simulink model "modelo_simulacao_Imagens_TCC"  (R2013a)
settings: Solver=ode3  StartTime=0.0  StopTime=1000  FixedStep=0.05  MaxStep=0.1  RelTol=1e-3
undefined symbols (not defined in the file): Dt, Ix, Iy, Iz, Mx, My, Mz, q0, q1, q2, q3, Ref_x, Ref_y, Ref_z, vax, vay, vaz, vnx, vny, vnz, vox, voy, voz, Vsx, Vsy, Vsz, Wx, Wy, Wz, X, Xref, Y, Yref, Z, Zref
libraries: vrlib x4, aerolibutil x3, aerolibtransform2 x2
settings Model: Creator=Daniel  LastModifiedBy=Daniel

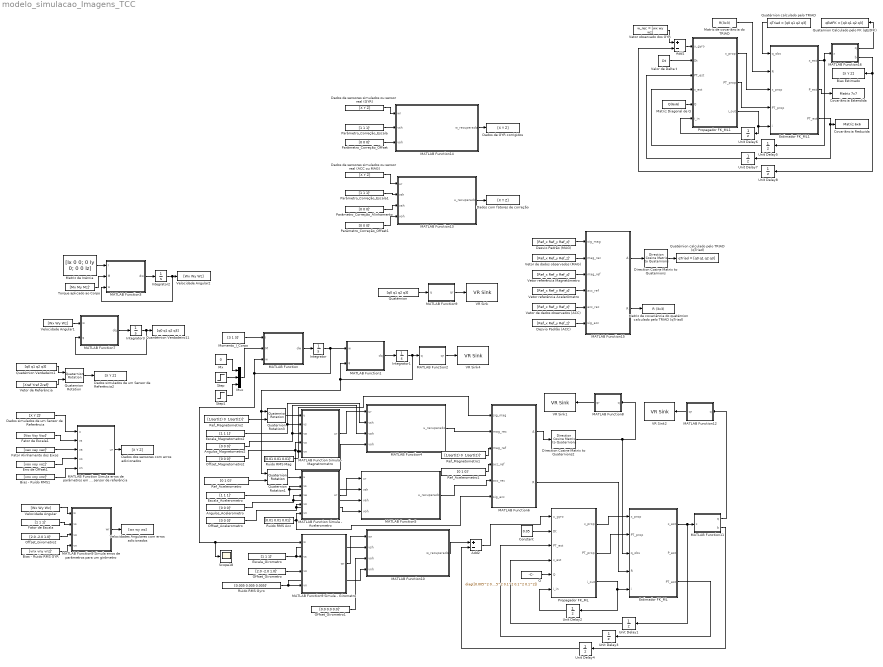
== system modelo_simulacao_Imagens_TCC ==
  Add1 : Sum  Inputs=+-
  Add2 : Sum  Inputs=+-
  Angulos_Acelerometro : Constant  Value=[0 0 0]'
  Angulos_Magnetometro2 : Constant  Value=[0 0 0]'
  Bias - Ruido RMS GYR : Constant  Value=[vnx vny vnz]'
  Bias - Ruído RMS1 : Constant  Value=[vnx vny vnz]'
  Bias Estimado : ToFile  Filename=[X Y Z]  SaveFormat=Timeseries
  Constant : Constant  Value=0.05
  Covariância Estendida : ToFile  Filename=Matriz 7x7  SaveFormat=Timeseries
  Covariância Reduzida : ToFile  Filename=Matriz 6x6  SaveFormat=Timeseries
  Dados com fatores de correção : ToFile  Filename=[X Y Z]  SaveFormat=Timeseries
  Dados de GYR corrigidos : ToFile  Filename=[X Y Z]  SaveFormat=Timeseries
  Dados de sensores simulados ou sensor real (ACC ou MAG) : Constant  Value=[X Y Z]
  Dados de sensores simulados ou sensor real (GYR) : Constant  Value=[X Y Z]
  Dados dos sensores com erros adicionados : ToFile  Filename=[X Y Z]  SaveFormat=Timeseries
  Dados simulados de um Sensor de Referência : Constant  Value=[X Y Z]'
  Dados simulados de um Sensor de Referência2 : ToFile  Filename=[X Y Z]  SaveFormat=Timeseries
  Desvio Padrão (ACC) : Constant  Value=[Ref_x Ref_y Ref_z]'
  Desvio Padrão (MAG) : Constant  Value=[Ref_x Ref_y Ref_z]'
  Direction Cosine Matrix to Quaternions : aerolibtransform2/Direction Cosine Matrix  to Quaternions
  Direction Cosine Matrix to Quaternions2 : aerolibtransform2/Direction Cosine Matrix  to Quaternions
  Erro de Offset1 : Constant  Value=[vox voy voz]'
  Escala_Acelerometro : Constant  Value=[1 1 1]'
  Escala_Girometro : Constant  Value=[1 1 1]'
  Escala_Magnetometro2 : Constant  Value=[1 1 1]'
  Estimador FK_ML : MATLAB Function  TreatAsAtomicUnit=on
  Estimador FK_ML1 : MATLAB Function  TreatAsAtomicUnit=on
  Fator Alinhamento dos Eixos : Constant  Value=[vax vay vaz]'
  Fator de Escala : Constant  Value=[1 1 1]'
  Fator de Escala1 : Constant  Value=[Vsx Vsy Vsz]'
  Integrator : Integrator  InitialCondition=[0 0 0]
  Integrator1 : Integrator  InitialCondition=[1 0 0 0]
  Integrator2 : Integrator  InitialCondition=[0 0 0]
  Integrator3 : Integrator  InitialCondition=[1 0 0 0]
  MATLAB Function : MATLAB Function  TreatAsAtomicUnit=on
  MATLAB Function Simula - Acelerometro : MATLAB Function  TreatAsAtomicUnit=on
  MATLAB Function Simula - Magnetrometro : MATLAB Function  TreatAsAtomicUnit=on
  MATLAB Function Simula erros de parâmetros em um sensor de referência : MATLAB Function  TreatAsAtomicUnit=on
  MATLAB Function1 : MATLAB Function  TreatAsAtomicUnit=on
  MATLAB Function10 : MATLAB Function  TreatAsAtomicUnit=on
  MATLAB Function11 : MATLAB Function  TreatAsAtomicUnit=on
  MATLAB Function12 : MATLAB Function  TreatAsAtomicUnit=on
  MATLAB Function13 : MATLAB Function  TreatAsAtomicUnit=on
  MATLAB Function14 : MATLAB Function  TreatAsAtomicUnit=on
  MATLAB Function15 : MATLAB Function  TreatAsAtomicUnit=on
  MATLAB Function16 : MATLAB Function  TreatAsAtomicUnit=on
  MATLAB Function2 : MATLAB Function  TreatAsAtomicUnit=on
  MATLAB Function3 : MATLAB Function  TreatAsAtomicUnit=on
  MATLAB Function4 : MATLAB Function  TreatAsAtomicUnit=on
  MATLAB Function5 : MATLAB Function  TreatAsAtomicUnit=on
  MATLAB Function6 : MATLAB Function  TreatAsAtomicUnit=on
  MATLAB Function7 : MATLAB Function  TreatAsAtomicUnit=on
  MATLAB Function8 : MATLAB Function  TreatAsAtomicUnit=on
  MATLAB Function9 : MATLAB Function  TreatAsAtomicUnit=on
  MATLAB Function9 Simula - Girometro : MATLAB Function  TreatAsAtomicUnit=on
  MATLAB Function9 Simula erros de parâmetros para um girômetro : MATLAB Function  TreatAsAtomicUnit=on
  Matriz Diagonal de Q : FromFile  FileName=Q(6x6)  SampleTime=0
  Matriz de Inércia : Constant  Value=[Ix 0 0; 0 Iy 0; 0 0 Iz]
  Matriz de covariância do quatérnion calculado pelo TRIAD (qTriad) : ToFile  Filename=R (3x3)  SaveFormat=Timeseries
  Matriz de covariância do TRIAD : FromFile  FileName=R(3x3)  SampleTime=0
  Momento_I_Corpo : Constant  Value=[3 1 3]'
  Mux : Mux  Inputs=3
  Mx : Constant  Value=0
  Offset_Acelerometro : Constant  Value=[0 0 0]'
  Offset_Girometro : Constant  Value=[2.0 -2.0 1.0]'
  Offset_Girometro1 : Constant  Value=[0.0 0.0 0.0]'
  Offset_Girometro2 : Constant  Value=[2.0 -2.0 1.0]'
  Offset_Magnetometro2 : Constant  Value=[0 0 0]'
  Parâmetro_Correção_Alinhamento : Constant  Value=[0 0 0]'
  Parâmetro_Correção_Escala : Constant  Value=[1 1 1]'
  Parâmetro_Correção_Escala1 : Constant  Value=[1 1 1]'
  Parâmetro_Correção_Offset : Constant  Value=[0 0 0]'
  Parâmetro_Correção_Offset1 : Constant  Value=[0 0 0]'
  Propagador FK_ML : MATLAB Function  TreatAsAtomicUnit=on
  Propagador FK_ML1 : MATLAB Function  TreatAsAtomicUnit=on
  Q : Constant  Value=diag([0.005^2 0.005^2 0.005^2 0.1^2 0.1^2 0.1^2])
  Quantérnion Verdadeiro11 : ToFile  Filename=[q0 q1 q2 q3]  SaveFormat=Timeseries
  Quaternion Rotation : aerolibutil/Quaternion Rotation
  Quaternion Rotation1 : aerolibutil/Quaternion Rotation
  Quaternion Rotation3 : aerolibutil/Quaternion Rotation
  Quaternion Calculado pelo FK (qEstFK) : ToFile  Filename=qEstFK = [q0 q1 q2 q3]  SaveFormat=Timeseries
  Quatérnion : Constant  Value=[q0 q1 q2 q3]
  Quatérnion Verdadeiro1 : Constant  Value=[q0 q1 q2 q3]
  Quatérnion calculado pelo TRIAD : FromFile  FileName=qTriad = [q0 q1 q2 q3]  SampleTime=0
  Quatérnion calculado pelo TRIAD (qTriad) : ToFile  Filename=qTriad = [q0 q1 q2 q3]  SaveFormat=Timeseries
  Ref_Acelerometro : Constant  Value=[0 1 0]'
  Ref_Acelerometro1 : Constant  Value=[0 1 0]'
  Ref_Magnetometro1 : Constant  Value="[1/sqrt(2) 0  1/sqrt(2)]'"
  Ref_Magnetometro2 : Constant  Value="[1/sqrt(2) 0  1/sqrt(2)]'"
  Ruido RMS Acc : Constant  Value=[0.01 0.01 0.01]'
  Ruido RMS Gyro : Constant  Value=[0.005 0.005 0.005]'
  Ruido RMS Mag : Constant  Value=[0.01 0.01 0.01]'
  Scope18 : Scope
      settings: YMin=-0.03  YMax=0.12  SaveName=ScopeData18  MaxDataPoints=50000
  Step : Step  Time=.1  Before=5  After=0  SampleTime=0
  Step1 : Step  Time=.1  Before=1  After=0  SampleTime=0
  Torque aplicado ao Corpo : Constant  Value=[Mx My Mz]'
  Unit Delay1 : UnitDelay  InitialCondition=[0 0 0 1 0 0 0]'  SampleTime=-1
  Unit Delay2 : UnitDelay  SampleTime=-1
  Unit Delay3 : UnitDelay  InitialCondition=diag([1 1 1 1 1 1])*1E6  SampleTime=-1
  Unit Delay4 : UnitDelay  InitialCondition=[0 0 0]'  SampleTime=-1
  Unit Delay5 : UnitDelay  InitialCondition=[0 0 0 1 0 0 0]'  SampleTime=-1
  Unit Delay6 : UnitDelay  SampleTime=-1
  Unit Delay7 : UnitDelay  InitialCondition=diag([1 1 1 1 1 1])*1E6  SampleTime=-1
  Unit Delay8 : UnitDelay  InitialCondition=[0 0 0]'  SampleTime=-1
  VR Sink : vrlib/VR Sink  InstantiateOnLoad=on  SampleTime=-1  ViewEnable=on  RemoteChange=off  RemoteView=off  FieldsWritten=H.rotation.4.1.1.double  WorldFileName=C:\Users\Administrator\Desktop\Arquivos WRL\cilindro3.wrl  AutoView=off  VideoDimensions=[]  AllowVariableSize=off
  VR Sink1 : vrlib/VR Sink  InstantiateOnLoad=on  SampleTime=-1  ViewEnable=on  RemoteChange=off  RemoteView=off  FieldsWritten=H.rotation.4.1.1.double  WorldFileName=C:\Users\Administrator\Desktop\Arquivos WRL\cilindro4.wrl  AutoView=off  VideoDimensions=[]  AllowVariableSize=off
  VR Sink2 : vrlib/VR Sink  InstantiateOnLoad=on  SampleTime=-1  ViewEnable=on  RemoteChange=off  RemoteView=off  FieldsWritten=H.rotation.4.1.1.double  WorldFileName=C:\Users\Administrator\Desktop\Arquivos WRL\cilindro5.wrl  AutoView=off  VideoDimensions=[]  AllowVariableSize=off
  VR Sink4 : vrlib/VR Sink  InstantiateOnLoad=on  SampleTime=-1  ViewEnable=on  RemoteChange=off  RemoteView=off  FieldsWritten=H.rotation.4.1.1.double  WorldFileName=C:\Users\Administrator\Desktop\Arquivos WRL\cilindro3.wrl  AutoView=off  VideoDimensions=[]  AllowVariableSize=off
  Valor de Delta t : Constant  Value=Dt
  Velocidade Angular : Constant  Value=[Wx Wy Wz]
  Velocidade Angular1 : Constant  Value=[Wx Wy Wz]
  Velocidade Angular2 : ToFile  Filename=[Wx Wy Wz]  SaveFormat=Timeseries
  Velocidades Angulares com erros adicionados : ToFile  Filename=[wx wy wz]  SaveFormat=Timeseries
  Vetor de Referência : Constant  Value=[Xref Yref Zref]'
  Vetor de dados observados (ACC) : Constant  Value=[Ref_x Ref_y Ref_z]'
  Vetor de dados observados (MAG) : Constant  Value=[Ref_x Ref_y Ref_z]'
  Vetor observado dos GYR : FromFile  FileName=w_rec = [wx wy wz]  SampleTime=0
  Vetor referência Acelerômetro : Constant  Value=[Ref_x Ref_y Ref_z]'
  Vetor referência Magnetômetro : Constant  Value=[Ref_x Ref_y Ref_z]'
  wires:
  Momento_I_Corpo/1 -> MATLAB Function/1(I)
  Mux/1 -> MATLAB Function/2(M)
  Mx/1 -> Mux/1
  Step/1 -> Mux/2
  Step1/1 -> Mux/3
  MATLAB Function/1(dw) -> Integrator/1
  Integrator/1 -> MATLAB Function1/1(w), MATLAB Function/3(w), Scope18/1, MATLAB Function9 Simula - Girometro/1(w)
  MATLAB Function1/1(dq) -> Integrator1/1
  MATLAB Function2/1(qr) -> VR Sink4/1
  Quaternion Rotation3/1 -> MATLAB Function Simula - Magnetrometro/1(u)
  Quaternion Rotation1/1 -> MATLAB Function Simula - Acelerometro/1(u)
  Ref_Magnetometro2/1 -> Quaternion Rotation3/2
  Ref_Acelerometro/1 -> Quaternion Rotation1/2
  Ruido RMS Mag/1 -> MATLAB Function6/1(sig_mag), MATLAB Function Simula - Magnetrometro/5(vn)
  Ruido RMS Acc/1 -> MATLAB Function Simula - Acelerometro/5(vn), MATLAB Function6/6(sig_acc)
  Offset_Magnetometro2/1 -> MATLAB Function Simula - Magnetrometro/4(vo), MATLAB Function4/4(voh)
  Escala_Acelerometro/1 -> MATLAB Function Simula - Acelerometro/2(vs), MATLAB Function5/2(vsh)
  Angulos_Acelerometro/1 -> MATLAB Function Simula - Acelerometro/3(va), MATLAB Function5/3(vah)
  Offset_Acelerometro/1 -> MATLAB Function Simula - Acelerometro/4(vo), MATLAB Function5/4(voh)
  MATLAB Function Simula - Magnetrometro/1(ur) -> MATLAB Function4/1(ur)
  MATLAB Function Simula - Acelerometro/1(ur) -> MATLAB Function5/1(ur)
  Escala_Magnetometro2/1 -> MATLAB Function Simula - Magnetrometro/2(vs), MATLAB Function4/2(vsh)
  Angulos_Magnetometro2/1 -> MATLAB Function Simula - Magnetrometro/3(va), MATLAB Function4/3(vah)
  MATLAB Function5/1(u_recuperado) -> MATLAB Function6/5(acc_rec)
  MATLAB Function4/1(u_recuperado) -> MATLAB Function6/2(mag_rec)
  Ref_Magnetometro1/1 -> MATLAB Function6/3(mag_ref)
  Ref_Acelerometro1/1 -> MATLAB Function6/4(acc_ref)
  MATLAB Function6/1(A) -> Direction Cosine Matrix to Quaternions2/1
  MATLAB Function8/1(qr) -> VR Sink1/1
  MATLAB Function9 Simula - Girometro/1(wr) -> MATLAB Function10/1(wr)
  Escala_Girometro/1 -> MATLAB Function10/2(vsh), MATLAB Function9 Simula - Girometro/2(vs)
  Offset_Girometro/1 -> MATLAB Function9 Simula - Girometro/3(vo)
  Ruido RMS Gyro/1 -> MATLAB Function10/4(vnh), MATLAB Function9 Simula - Girometro/4(vn)
  Offset_Girometro1/1 -> MATLAB Function10/3(voh)
  Propagador FK_ML/1(x_prop) -> Estimador FK_ML/1(x_prop)
  Propagador FK_ML/3(i_out) -> Unit Delay2/1, Estimador FK_ML/5(i)
  Unit Delay2/1 -> Propagador FK_ML/6(i_in)
  Q/1 -> Propagador FK_ML/5(Q)
  Constant/1 -> Propagador FK_ML/2(Dt)
  MATLAB Function10/1(w_recuperado) -> Add2/1
  MATLAB Function6/2(R) -> Estimador FK_ML/4(R)
  Estimador FK_ML/3(PT_est) -> Unit Delay3/1
  Unit Delay1/1 -> Propagador FK_ML/4(x_est)
  Unit Delay3/1 -> Propagador FK_ML/3(PT_est)
  Propagador FK_ML/2(PT_prop) -> Estimador FK_ML/2(PT_prop)
  Direction Cosine Matrix to Quaternions2/1 -> MATLAB Function8/1(q), Estimador FK_ML/3(q_obs)
  Integrator1/1 -> Quaternion Rotation3/1, Quaternion Rotation1/1, MATLAB Function1/2(q), MATLAB Function2/1(q)
  Estimador FK_ML/1(x_est) -> Unit Delay1/1, MATLAB Function11/1(x)
  Add2/1 -> Propagador FK_ML/1(u_gyro)
  MATLAB Function11/2(b) -> Unit Delay4/1
  Unit Delay4/1 -> Add2/2
  MATLAB Function12/1(qr) -> VR Sink2/1
  MATLAB Function11/1(q) -> MATLAB Function12/1(q)
  MATLAB Function3/1(dw) -> Integrator2/1
  Integrator2/1 -> Velocidade Angular2/1, MATLAB Function3/3(w)
  Matriz de Inércia/1 -> MATLAB Function3/1(I)
  Torque aplicado ao Corpo/1 -> MATLAB Function3/2(M)
  MATLAB Function7/1(dq) -> Integrator3/1
  Integrator3/1 -> Quantérnion Verdadeiro11/1, MATLAB Function7/2(q)
  Velocidade Angular1/1 -> MATLAB Function7/1(w)
  Vetor de Referência/1 -> Quaternion Rotation/2
  Quatérnion Verdadeiro1/1 -> Quaternion Rotation/1
  Quaternion Rotation/1 -> Dados simulados de um Sensor de Referência2/1
  Fator de Escala1/1 -> MATLAB Function Simula erros de parâmetros em um sensor de referência/2(vs)
  Fator Alinhamento dos Eixos/1 -> MATLAB Function Simula erros de parâmetros em um sensor de referência/3(va)
  Erro de Offset1/1 -> MATLAB Function Simula erros de parâmetros em um sensor de referência/4(vo)
  Bias - Ruído RMS1/1 -> MATLAB Function Simula erros de parâmetros em um sensor de referência/5(vn)
  Dados simulados de um Sensor de Referência/1 -> MATLAB Function Simula erros de parâmetros em um sensor de referência/1(u)
  MATLAB Function Simula erros de parâmetros em um sensor de referência/1(ur) -> Dados dos sensores com erros adicionados/1
  Bias - Ruido RMS GYR/1 -> MATLAB Function9 Simula erros de parâmetros para um girômetro/4(vn)
  Fator de Escala/1 -> MATLAB Function9 Simula erros de parâmetros para um girômetro/2(vs)
  Offset_Girometro2/1 -> MATLAB Function9 Simula erros de parâmetros para um girômetro/3(vo)
  MATLAB Function9 Simula erros de parâmetros para um girômetro/1(wr) -> Velocidades Angulares com erros adicionados/1
  Velocidade Angular/1 -> MATLAB Function9 Simula erros de parâmetros para um girômetro/1(w)
  MATLAB Function9/1(qr) -> VR Sink/1
  Quatérnion/1 -> MATLAB Function9/1(q)
  Parâmetro_Correção_Escala1/1 -> MATLAB Function13/2(vsh)
  Parâmetro_Correção_Alinhamento/1 -> MATLAB Function13/3(vah)
  Parâmetro_Correção_Offset1/1 -> MATLAB Function13/4(voh)
  Dados de sensores simulados ou sensor real (ACC ou MAG)/1 -> MATLAB Function13/1(ur)
  MATLAB Function13/1(u_recuperado) -> Dados com fatores de correção/1
  MATLAB Function14/1(w_recuperado) -> Dados de GYR corrigidos/1
  Parâmetro_Correção_Offset/1 -> MATLAB Function14/3(voh)
  Parâmetro_Correção_Escala/1 -> MATLAB Function14/2(vsh)
  Dados de sensores simulados ou sensor real (GYR)/1 -> MATLAB Function14/1(wr)
  MATLAB Function15/1(A) -> Direction Cosine Matrix to Quaternions/1
  Vetor referência Acelerômetro/1 -> MATLAB Function15/4(acc_ref)
  Vetor referência Magnetômetro/1 -> MATLAB Function15/3(mag_ref)
  Vetor de dados observados (ACC)/1 -> MATLAB Function15/5(acc_rec)
  Desvio Padrão (ACC)/1 -> MATLAB Function15/6(sig_acc)
  Desvio Padrão (MAG)/1 -> MATLAB Function15/1(sig_mag)
  Vetor de dados observados (MAG)/1 -> MATLAB Function15/2(mag_rec)
  Direction Cosine Matrix to Quaternions/1 -> Quatérnion calculado pelo TRIAD (qTriad)/1
  MATLAB Function15/2(R) -> Matriz de covariância do quatérnion calculado pelo TRIAD (qTriad)/1
  Propagador FK_ML1/1(x_prop) -> Estimador FK_ML1/3(x_prop)
  Propagador FK_ML1/3(i_out) -> Unit Delay6/1, Estimador FK_ML1/5(i)
  Unit Delay6/1 -> Propagador FK_ML1/6(i_in)
  Valor de Delta t/1 -> Propagador FK_ML1/2(Dt)
  Estimador FK_ML1/3(PT_est) -> Covariância Reduzida/1, Unit Delay7/1
  Unit Delay5/1 -> Propagador FK_ML1/4(x_est)
  Unit Delay7/1 -> Propagador FK_ML1/3(PT_est)
  Propagador FK_ML1/2(PT_prop) -> Estimador FK_ML1/4(PT_prop)
  Estimador FK_ML1/1(x_est) -> MATLAB Function16/1(x), Unit Delay5/1
  Add1/1 -> Propagador FK_ML1/1(u_gyro)
  MATLAB Function16/2(b) -> Bias Estimado/1, Unit Delay8/1
  Unit Delay8/1 -> Add1/2
  MATLAB Function16/1(q) -> Quaternion Calculado pelo FK (qEstFK)/1
  Estimador FK_ML1/2(P_est) -> Covariância Estendida/1
  Matriz Diagonal de Q/1 -> Propagador FK_ML1/5(Q)
  Matriz de covariância do TRIAD/1 -> Estimador FK_ML1/2(R)
  Quatérnion calculado pelo TRIAD/1 -> Estimador FK_ML1/1(q_obs)
  Vetor observado dos GYR/1 -> Add1/1

== matlab function modelo_simulacao_Imagens_TCC/MATLAB Function1 ==
  data: w input; dq output; q input
function dq = cinematica(w,q)
%#eml
wx = w(1);
wy = w(2);
wz = w(3);

q = q/norm(q);

qteta = q(1);
qx = q(2);
qy = q(3);
qz = q(4);

W = [0 -wx -wy -wz; wx 0 wz -wy; wy -wz 0 wx; wz wy -wx 0];
%W=[0 wz -wy wx; -wz 0 wx wy; wy -wx 0 wz; -wx -wy -wz 0];
dq=0.5*W*[qteta qx qy qz]';

== matlab function modelo_simulacao_Imagens_TCC/MATLAB Function ==
  data: I input; dw output; M input; w input
function dw  = Eq_Euler(I,M,w)
%#eml
wx = w(1);
wy = w(2);
wz = w(3);

Ix = I(1);
Iy = I(2);
Iz = I(3);

Mx = M(1);
My = M(2);
Mz = M(3);

dwx = (Mx - wy*wz*(Iz - Iy))/Ix;
dwy = (My - wx*wz*(Ix - Iz))/Iy;
dwz = (Mz - wx*wy*(Iy - Ix))/Iz;

dw=[dwx dwy dwz]';

== matlab function modelo_simulacao_Imagens_TCC/MATLAB Function2 ==
  data: q input; qr output
function qr = ajusta_q(q)
%#eml

q = q/(norm(q));
v = [q(2) q(3) q(4)] / norm([q(2) q(3) q(4)]);
ang = acos(q(1))*2;

qr = [v ang];

== matlab function modelo_simulacao_Imagens_TCC/MATLAB Function3 ==
  data: I input; dw output; M input; w input
function dw  = Eq_Euler(I,M,w)
%#eml
wx = w(1);
wy = w(2);
wz = w(3);

Ix = I(1);
Iy = I(2);
Iz = I(3);

Mx = M(1);
My = M(2);
Mz = M(3);

dwx = (Mx - wy*wz*(Iz - Iy))/Ix;
dwy = (My - wx*wz*(Ix - Iz))/Iy;
dwz = (Mz - wx*wy*(Iy - Ix))/Iz;

dw=[dwx dwy dwz]';

== matlab function modelo_simulacao_Imagens_TCC/MATLAB Function Simula - Magnetrometro ==
  data: u input; ur output; vs input; va input; vo input; vn input
function ur = triad_model(u,vs,va,vo,vn)
%#eml

rho = va(1);
phi = va(2);
lambda = va(3);

S = diag(vs);
T = [1 0 0; sin(rho) cos(rho) 0;...
    sin(phi)*cos(lambda) sin(lambda)*cos(phi) cos(phi)*cos(lambda)];

ur = S*T*u + vo + vn.*randn(3,1);

== matlab function modelo_simulacao_Imagens_TCC/MATLAB Function Simula - Acelerometro ==
  data: u input; ur output; vs input; va input; vo input; vn input
function ur = triad_model(u,vs,va,vo,vn)
%#eml

rho = va(1);
phi = va(2);
lambda = va(3);

S = diag(vs);
T = [1 0 0; sin(rho) cos(rho) 0;...
    sin(phi)*cos(lambda) sin(lambda)*cos(phi) cos(phi)*cos(lambda)];

ur = S*T*u + vo + vn.*randn(3,1);

== matlab function modelo_simulacao_Imagens_TCC/MATLAB Function4 ==
  data: ur input; u_recuperado output; vsh input; vah input; voh input
function u_recuperado = inv_triad_model(ur,vsh,vah,voh)
%#eml

rho = vah(1);
phi = vah(2);
lambda = vah(3);

T_inv = [1 0 0; -tan(rho) 1/cos(rho) 0;...
    tan(rho)*tan(lambda)-tan(phi) -tan(lambda)/cos(rho) 1/(cos(lambda)*cos(phi))];
S_inv = inv(diag(vsh));

u_recuperado = T_inv*S_inv*(ur - voh);

== matlab function modelo_simulacao_Imagens_TCC/MATLAB Function5 ==
  data: ur input; u_recuperado output; vsh input; vah input; voh input
function u_recuperado = inv_triad_model(ur,vsh,vah,voh)
%#eml

rho = vah(1);
phi = vah(2);
lambda = vah(3);

T_inv = [1 0 0; -tan(rho) 1/cos(rho) 0;...
    tan(rho)*tan(lambda)-tan(phi) -tan(lambda)/cos(rho) 1/(cos(lambda)*cos(phi))];
S_inv = inv(diag(vsh));

u_recuperado = T_inv*S_inv*(ur - voh);

== matlab function modelo_simulacao_Imagens_TCC/MATLAB Function6 ==
  data: sig_mag input; A output; mag_rec input; mag_ref input; acc_ref input; acc_rec input; sig_acc input; R output
function [A,R] = TRIAD(sig_mag,mag_rec,mag_ref,acc_ref,acc_rec,sig_acc)

% ========== Função de Determinação de Atitude ===========
% ========== Algoritmo TRIAD ===========
% Os parâmetros de Entrada são:
% V1 : vetor de referência V1
V1 = acc_ref;
% V2 : vetor de referência V2
V2 = mag_ref;
% W1 : vetor de observação W1
W1 = acc_rec;
% W2 : vetor de observação W2
W2 = mag_rec;
% SigTo1 : desvio padrão das observação do Acelerômetro
SigTot1 = sig_acc(1);
% SigTo2 : desvio padrão das observação do Magnetômetro
SigTot2 = sig_mag(1);

% ========================================================
% Os parâmetros de Retorno são:
% A : matriz de atitude
% P : Covariância da atitude
% ========================================================
% --- Obtendo a Tríade de Referência
r1 = V1/norm(V1);
r2 = cross(V1,V2); % função do produto vetorial
r2 = r2 / norm(r2);
r3 = cross(r1,r2);
% --- Montando a Matriz de Referência
Mref = [r1 r2 r3];
% --- Obtendo a tríade de observação
s1 = W1/norm(W1);
s2 = cross(W1,W2);
s2 = s2 / norm(s2);
s3 = cross(s1,s2);
% --- Montando a Matriz de Observação
Mobs = [s1 s2 s3];
% --- Atitude pelo TRIAD
A = Mobs * Mref';
%--------------------------------------------------------------------------
% Obtendo a covariância da atitude (P = P + AP AT)
R = SigTot1^2 * eye(3) + ...
    (1/norm(cross(W1,W2)))^2 * (SigTot1^2* (W1'*W2) * (W1*W2' + W2*W1')...
    + (SigTot2^2 - SigTot1^2)*W1*W1');

%--------------------------------------------------------------------------

== matlab function modelo_simulacao_Imagens_TCC/MATLAB Function7 ==
  data: w input; dq output; q input
function dq = cinematica(w,q)
%#eml
wx = w(1);
wy = w(2);
wz = w(3);

q = q/norm(q);

qteta = q(1);
qx = q(2);
qy = q(3);
qz = q(4);

W = [0 -wx -wy -wz; wx 0 wz -wy; wy -wz 0 wx; wz wy -wx 0];
%W=[0 wz -wy wx; -wz 0 wx wy; wy -wx 0 wz; -wx -wy -wz 0];
dq=0.5*W*[qteta qx qy qz]';

== matlab function modelo_simulacao_Imagens_TCC/MATLAB Function8 ==
  data: q input; qr output
function qr = ajusta_q(q)
%#eml

q = q/(norm(q));
v = [q(2) q(3) q(4)] / norm([q(2) q(3) q(4)]);
ang = acos(q(1))*2;

qr = [v ang];

== matlab function modelo_simulacao_Imagens_TCC/MATLAB Function9 Simula - Girometro ==
  data: w input; wr output; vs input; vo input; vn input
function wr = gyro_model(w,vs,vo,vn)
%#eml

S = diag(vs);

wr = S*w + vo + vn.*randn(3,1);

== matlab function modelo_simulacao_Imagens_TCC/MATLAB Function10 ==
  data: wr input; w_recuperado output; vsh input; voh input; vnh input
function w_recuperado = inv_gyro_model(wr,vsh,voh,vnh)
%#eml

S_inv = inv(diag(vsh));

w_recuperado = S_inv*(wr - voh);

== matlab function modelo_simulacao_Imagens_TCC/MATLAB Function Simula erros de parâmetros em um sensor de referência ==
  data: u input; ur output; vs input; va input; vo input; vn input
function ur = sensor_model(u,vs,va,vo,vn)

rho = va(1);
phi = va(2);
lambda = va(3);

S = diag(vs);
T = [1 0 0; sin(rho) cos(rho) 0;...
    sin(phi)*cos(lambda) sin(lambda)*cos(phi) cos(phi)*cos(lambda)];

ur = S*T*u + vo + vn.*randn(3,1);

== matlab function modelo_simulacao_Imagens_TCC/MATLAB Function11 ==
  data: x input; q output; b output
function [q,b] = separa(x)
q = [x(4,1); x(1:3,1)];
b = x(5:7,1);
end

== matlab function modelo_simulacao_Imagens_TCC/MATLAB Function12 ==
  data: q input; qr output
function qr = ajusta_q(q)
%#eml

q = q/(norm(q));
v = [q(2) q(3) q(4)] / norm([q(2) q(3) q(4)]);
ang = acos(q(1))*2;

qr = [v ang];

== matlab function modelo_simulacao_Imagens_TCC/MATLAB Function9 Simula erros de parâmetros para um girômetro ==
  data: w input; wr output; vs input; vo input; vn input
function wr = gyro_model(w,vs,vo,vn)

S = diag(vs);
wr = S*w + vo + vn.*randn(3,1);

== matlab function modelo_simulacao_Imagens_TCC/MATLAB Function9 ==
  data: q input; qr output
function qr = ajusta_q(q)
%#eml

q = q/(norm(q));
v = [q(2) q(3) q(4)] / norm([q(2) q(3) q(4)]);
ang = acos(q(1))*2;

qr = [v ang];

== matlab function modelo_simulacao_Imagens_TCC/Propagador FK_ML ==
  data: u_gyro input; x_prop output; Dt input; PT_est input; x_est input; Q input; PT_prop output; i_in input; i_out output
function [x_prop, PT_prop, i_out] = propagador_FK(u_gyro, Dt, PT_est, x_est, Q, i_in)
%#codegen

i_out = i_in + 1;

% ================== Propagação ==================
% ------ Propagação do Estado
% São medidos os Girômetros e sua saída subtraida
% do bias é integrada no período de propagação

q_est = x_est(1:4,1);
b_est = x_est(5:7,1);


% Matriz de atualização do quaternion
Th = u_gyro * Dt;

Omega4 = [ 0     Th(3) -Th(2)  Th(1);
	  -Th(3)  0     Th(1)  Th(2); 
      Th(2) -Th(1)  0     Th(3);
     -Th(1) -Th(2) -Th(3)  0   ];

M = eye(4) * cos(norm(Th)/2) + Omega4 * sin(norm(Th)/2) / norm(Th);
q_prop = M * q_est; 

b_prop = b_est;

x_prop = [q_prop ; b_prop];

% Matriz Constante // A ser executado fora dessa função
GT = [ -1/2*eye(3) zeros(3,3); zeros(3,3) eye(3)];
QT = GT * Q * GT';

% ---------------------

Omega3_prop = [ 0     q_prop(3) -q_prop(2);
	  -q_prop(3)  0     q_prop(1); 
      q_prop(2) -q_prop(1)  0   ];

A_prop = (q_prop(4)^2 - norm(q_prop(1:3,1))^2)*eye(3) + 2*q_prop(1:3,1)*q_prop(1:3,1)' ... 
      + 2*q_prop(4)*Omega3_prop;
  
Omega3_est = [ 0     q_est(3) -q_est(2);
	  -q_est(3)  0     q_est(1); 
      q_est(2) -q_est(1)  0   ];  
  
A_est = (q_est(4)^2 - norm(q_est(1:3,1))^2)*eye(3) + 2*q_est(1:3,1)*q_est(1:3,1)' ... 
      + 2*q_est(4)*Omega3_est;
  
% ------ Propagação da Matriz de Covariância
L = A_prop * A_est';
KK = -1/2 * (L + eye(3)) * Dt/2;  % Integral Trapézio
PhiT = [L KK; zeros(3,3) eye(3)];
SiG = (PhiT * QT * PhiT' + QT) * Dt/2; % Integral Trapézio
PT_prop = PhiT * PT_est * PhiT' + SiG;

== matlab function modelo_simulacao_Imagens_TCC/MATLAB Function13 ==
  data: ur input; u_recuperado output; vsh input; vah input; voh input
function u_recuperado = inv_sensor_model(ur,vsh,vah,voh)

rho = vah(1);
phi = vah(2);
lambda = vah(3);

T_inv = [1 0 0; -tan(rho) 1/cos(rho) 0;...
    tan(rho)*tan(lambda)-tan(phi) -tan(lambda)/cos(rho) 1/(cos(lambda)*cos(phi))];
S_inv = inv(diag(vsh));

u_recuperado = T_inv*S_inv*(ur - voh);

== matlab function modelo_simulacao_Imagens_TCC/Estimador FK_ML ==
  data: x_prop input size=7; x_est output size=7; PT_prop input size=[6,6]; q_obs input; R input; P_est output; PT_est output size=[6,6]; i input
function [x_est, P_est, PT_est] = Estimador_FK(x_prop, PT_prop, q_obs, R, i)

q = q_obs;
q_obs = [q(2); q(3); q(4); q(1)];

% ---- Separando as compoentes do estado
q_prop = x_prop(1:4,1);
b_prop = x_prop(5:7,1);


% ---- Montando a matriz E (Ksi)
E = [ q_prop(4) -q_prop(3)  q_prop(2);
      q_prop(3)  q_prop(4) -q_prop(1);
     -q_prop(2)  q_prop(1)  q_prop(4);
     -q_prop(1) -q_prop(2) -q_prop(3)];

% ---- Montando a matriz S
S  = [E zeros(4,3); zeros(3,3) eye(3)];

if (mod(i,2) ~= 0)    
    x_est = x_prop;
    PT_est = PT_prop;
    P_est   = S * PT_est * S';
else
    
% ---- Montando a matriz H e HT.
H  = [eye(4) zeros(4,3)];
HT = [E zeros(4,3)];

% ---- Separando covariancias dos estados
Ptt_prop = PT_prop(1:3,1:3);
Pbt_prop = PT_prop(4:6,1:3);

% ---- Cálculo do novo ganho (reduzido)
KT       = [Ptt_prop; Pbt_prop] * inv(Ptt_prop + R) * E';
% KT       = [Ptt_prop; Pbt_prop] * E' * inv(E*(Ptt_prop + P_Tri)*E');

    
% ---- Atualização da covariância reduzida
PT_est  = PT_prop - KT * HT * PT_prop; 

% ---- Cálculo da covariância estendida
P_est   = S * PT_est * S' ;

% ---- Cálculo do ganho estendido 
K        = S * KT;

% ---- Atualização do estado
if(dot(q_prop,q_obs) > 0)
    q_obs = q_obs;
else
    q_obs = -q_obs;
end

x_est   = x_prop + K * (q_obs - q_prop);

% ---- renormalização do quaternion
n = norm(x_est(1:4));           % norma do quatérnio
x_est(1:4,1) = x_est(1:4,1) / n; % renormalização do quaternion

end

== matlab function modelo_simulacao_Imagens_TCC/MATLAB Function14 ==
  data: wr input; w_recuperado output; vsh input; voh input
function w_recuperado = inv_gyro_model(wr,vsh,voh)

S_inv = inv(diag(vsh));
w_recuperado = S_inv*(wr - voh);

== matlab function modelo_simulacao_Imagens_TCC/MATLAB Function15 ==
  data: sig_mag input; A output; mag_rec input; mag_ref input; acc_ref input; acc_rec input; sig_acc input; R output
function [A,R] = TRIAD(sig_mag,mag_rec,mag_ref,acc_ref,acc_rec,sig_acc)

% ========== Função de Determinação de Atitude ===========
% ========== Algoritmo TRIAD ===========
% Os parâmetros de Entrada são:
% V1 : vetor de referência V1
V1 = acc_ref;
% V2 : vetor de referência V2
V2 = mag_ref;
% W1 : vetor de observação W1
W1 = acc_rec;
% W2 : vetor de observação W2
W2 = mag_rec;
% SigTo1 : desvio padrão das observação do Acelerômetro
SigTot1 = sig_acc(1);
% SigTo2 : desvio padrão das observação do Magnetômetro
SigTot2 = sig_mag(1);

% ========================================================
% Os parâmetros de Retorno são:
% A : matriz de atitude
% P : Covariância da atitude
% ========================================================
% --- Obtendo a Tríade de Referência
r1 = V1/norm(V1);
r2 = cross(V1,V2); % função do produto vetorial
r2 = r2 / norm(r2);
r3 = cross(r1,r2);
% --- Montando a Matriz de Referência
Mref = [r1 r2 r3];
% --- Obtendo a tríade de observação
s1 = W1/norm(W1);
s2 = cross(W1,W2);
s2 = s2 / norm(s2);
s3 = cross(s1,s2);
% --- Montando a Matriz de Observação
Mobs = [s1 s2 s3];
% --- Atitude pelo TRIAD
A = Mobs * Mref';
%--------------------------------------------------------------------------
% Obtendo a covariância da atitude (P = P + AP AT)
R = SigTot1^2 * eye(3) + ...
    (1/norm(cross(W1,W2)))^2 * (SigTot1^2* (W1'*W2) * (W1*W2' + W2*W1')...
    + (SigTot2^2 - SigTot1^2)*W1*W1');

%--------------------------------------------------------------------------

== matlab function modelo_simulacao_Imagens_TCC/Estimador FK_ML1 ==
  data: q_obs input; R input; x_prop input size=7; x_est output size=7; PT_prop input size=[6,6]; P_est output; PT_est output size=[6,6]; i input
function [x_est, P_est, PT_est] = Estimador_FK(q_obs, R, x_prop, PT_prop,  i)

q = q_obs;
q_obs = [q(2); q(3); q(4); q(1)];

% ---- Separando as compoentes do estado
q_prop = x_prop(1:4,1);
b_prop = x_prop(5:7,1);


% ---- Montando a matriz E (Ksi)
E = [ q_prop(4) -q_prop(3)  q_prop(2);
      q_prop(3)  q_prop(4) -q_prop(1);
     -q_prop(2)  q_prop(1)  q_prop(4);
     -q_prop(1) -q_prop(2) -q_prop(3)];

% ---- Montando a matriz S
S  = [E zeros(4,3); zeros(3,3) eye(3)];

if (mod(i,2) ~= 0)    
    x_est = x_prop;
    PT_est = PT_prop;
    P_est   = S * PT_est * S';
else
    
% ---- Montando a matriz H e HT.
H  = [eye(4) zeros(4,3)];
HT = [E zeros(4,3)];

% ---- Separando covariancias dos estados
Ptt_prop = PT_prop(1:3,1:3);
Pbt_prop = PT_prop(4:6,1:3);

% ---- Cálculo do novo ganho (reduzido)
KT       = [Ptt_prop; Pbt_prop] * inv(Ptt_prop + R) * E';
% KT       = [Ptt_prop; Pbt_prop] * E' * inv(E*(Ptt_prop + P_Tri)*E');

    
% ---- Atualização da covariância reduzida
PT_est  = PT_prop - KT * HT * PT_prop; 

% ---- Cálculo da covariância estendida
P_est   = S * PT_est * S' ;

% ---- Cálculo do ganho estendido 
K        = S * KT;

% ---- Atualização do estado
if(dot(q_prop,q_obs) > 0)
    q_obs = q_obs;
else
    q_obs = -q_obs;
end

x_est   = x_prop + K * (q_obs - q_prop);

% ---- renormalização do quaternion
n = norm(x_est(1:4));           % norma do quatérnio
x_est(1:4,1) = x_est(1:4,1) / n; % renormalização do quaternion

end

== matlab function modelo_simulacao_Imagens_TCC/MATLAB Function16 ==
  data: x input; q output; b output
function [q,b] = separa(x)
q = [x(4,1); x(1:3,1)];
b = x(5:7,1);
end

== matlab function modelo_simulacao_Imagens_TCC/Propagador FK_ML1 ==
  data: u_gyro input; x_prop output; Dt input; PT_est input; x_est input; Q input; PT_prop output; i_in input; i_out output
function [x_prop, PT_prop, i_out] = propagador_FK(u_gyro, Dt, PT_est, x_est, Q, i_in)
%#codegen

i_out = i_in + 1;

% ================== Propagação ==================
% ------ Propagação do Estado
% São medidos os Girômetros e sua saída subtraida
% do bias é integrada no período de propagação

q_est = x_est(1:4,1);
b_est = x_est(5:7,1);


% Matriz de atualização do quaternion
Th = u_gyro * Dt;

Omega4 = [ 0     Th(3) -Th(2)  Th(1);
	  -Th(3)  0     Th(1)  Th(2); 
      Th(2) -Th(1)  0     Th(3);
     -Th(1) -Th(2) -Th(3)  0   ];

M = eye(4) * cos(norm(Th)/2) + Omega4 * sin(norm(Th)/2) / norm(Th);
q_prop = M * q_est; 

b_prop = b_est;

x_prop = [q_prop ; b_prop];

% Matriz Constante // A ser executado fora dessa função
GT = [ -1/2*eye(3) zeros(3,3); zeros(3,3) eye(3)];
QT = GT * Q * GT';

% ---------------------

Omega3_prop = [ 0     q_prop(3) -q_prop(2);
	  -q_prop(3)  0     q_prop(1); 
      q_prop(2) -q_prop(1)  0   ];

A_prop = (q_prop(4)^2 - norm(q_prop(1:3,1))^2)*eye(3) + 2*q_prop(1:3,1)*q_prop(1:3,1)' ... 
      + 2*q_prop(4)*Omega3_prop;
  
Omega3_est = [ 0     q_est(3) -q_est(2);
	  -q_est(3)  0     q_est(1); 
      q_est(2) -q_est(1)  0   ];  
  
A_est = (q_est(4)^2 - norm(q_est(1:3,1))^2)*eye(3) + 2*q_est(1:3,1)*q_est(1:3,1)' ... 
      + 2*q_est(4)*Omega3_est;
  
% ------ Propagação da Matriz de Covariância
L = A_prop * A_est';
KK = -1/2 * (L + eye(3)) * Dt/2;  % Integral Trapézio
PhiT = [L KK; zeros(3,3) eye(3)];
SiG = (PhiT * QT * PhiT' + QT) * Dt/2; % Integral Trapézio
PT_prop = PhiT * PT_est * PhiT' + SiG;
